simulink model "Lab_2"  (R2017b)
settings: Solver=ode45  StartTime=0.0  StopTime=50  RelTol=1e-10
values from neighbouring files (symbols this model uses):
  I_1 = M/12 * (w^2 + l^2)    (= 0.0153029225)    [main.m]
  I_2 = M/12 * (w^2 + h^2)    (= 0.0314850625)    [main.m]
  I_3 = M/12 * (l^2 + h^2)    (= 0.041787985)    [main.m]
undefined symbols (not defined in the file or in its folder): DCM_0, phi_0, psi_0, theta_0
libraries: sharedutil x1
settings Model: Creator=fcuzzocrea  LastModifiedBy=fcuzzocrea

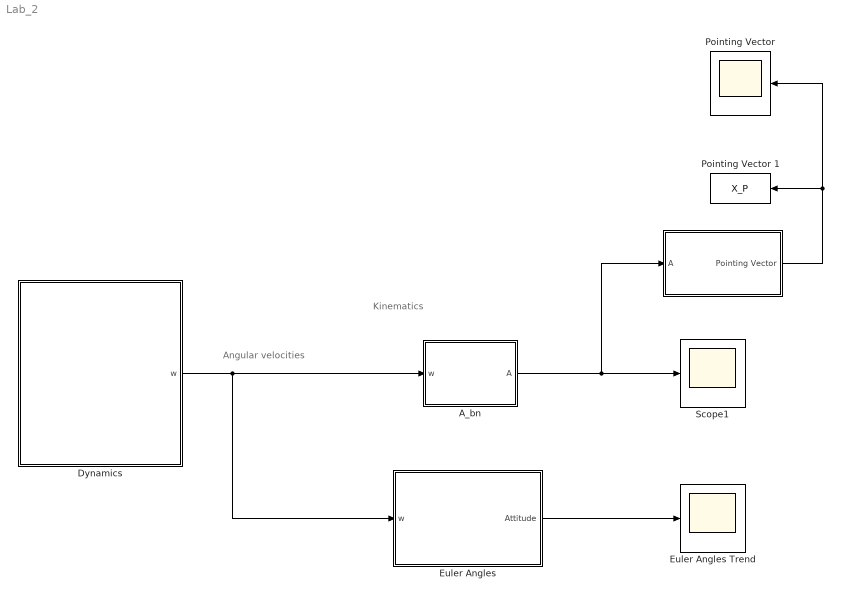
== system Lab_2 ==
  note: Kinematics
  note: Angular velocities
  " " : Subsystem
  A_bn : Subsystem
  "Dynamics " : Subsystem
  "Euler Angles " : Subsystem
  "Euler Angles Trend " : Scope
  Pointing Vector : Scope
  Pointing Vector 1 : ToWorkspace  VariableName=X_P  SampleTime=-1
  Scope1 : Scope
  wires:
  A_bn/1(A) -> " "/1(A), Scope1/1
  "Euler Angles "/1(Attitude) -> "Euler Angles Trend "/1
  "Dynamics "/1(w) -> "Euler Angles "/1(w), A_bn/1(w)
  " "/1("Pointing Vector ") -> Pointing Vector/1, Pointing Vector 1/1

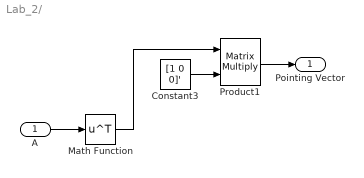
== system Lab_2/  ==
  A : Inport
  Constant3 : Constant  Value=[1 0 0]'  VectorParams1D=off
  Math Function : Math  Operator=transpose  SaturateOnIntegerOverflow=on
  Product1 : Product  Multiplication=Matrix(*)
  "Pointing Vector " : Outport
  wires:
  Constant3/1 -> Product1/2
  Math Function/1 -> Product1/1
  A/1 -> Math Function/1
  Product1/1 -> "Pointing Vector "/1

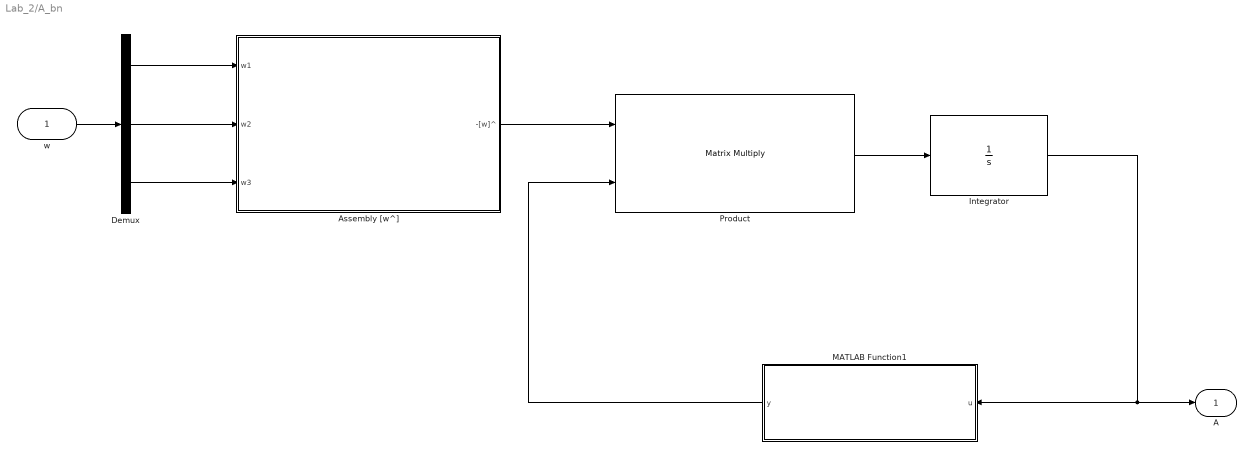
== system Lab_2/A_bn ==
  w : Inport  Unit=rad/s  PortDimensions=3
  "Assembly [w^] " : Subsystem
  Demux : Demux  Outputs=3
  Integrator : Integrator  InitialCondition=DCM_0
  MATLAB Function1 : MATLAB Function  TreatAsAtomicUnit=on
  Product : Product  Multiplication=Matrix(*)
  A : Outport
  wires:
  Product/1 -> Integrator/1
  Integrator/1 -> A/1, MATLAB Function1/1(u)
  w/1 -> Demux/1
  Demux/1 -> "Assembly [w^] "/1(w1)
  Demux/2 -> "Assembly [w^] "/2(w2)
  Demux/3 -> "Assembly [w^] "/3(w3)
  "Assembly [w^] "/1(-[w]^) -> Product/1
  MATLAB Function1/1(y) -> Product/2

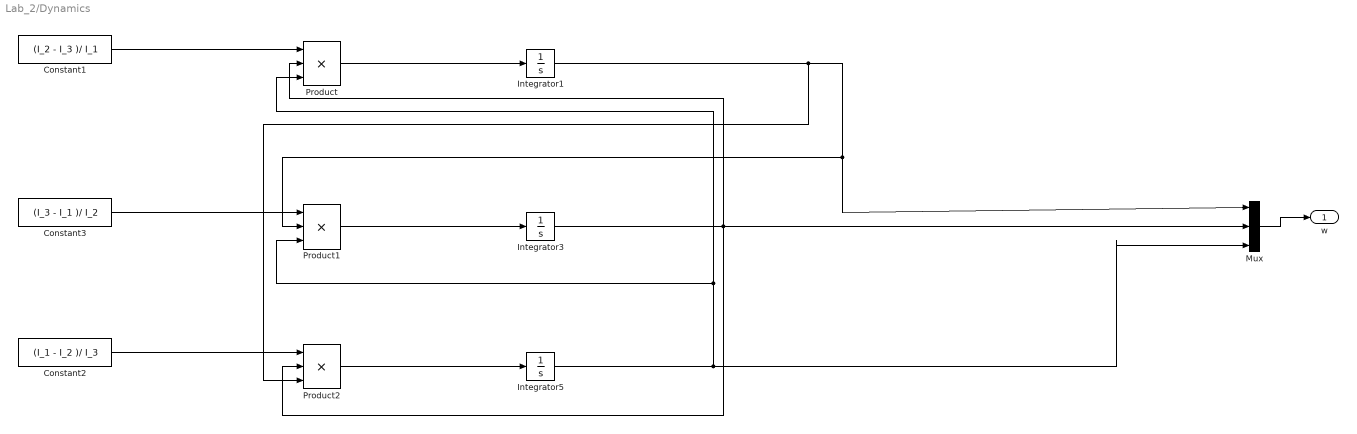
== system Lab_2/Dynamics  ==
  Constant1 : Constant  Value=(I_2 - I_3 )/ I_1
  Constant2 : Constant  Value=(I_1 - I_2 )/ I_3
  Constant3 : Constant  Value=(I_3 - I_1 )/ I_2
  Integrator1 : Integrator
  Integrator3 : Integrator  InitialCondition=0.45
  Integrator5 : Integrator  InitialCondition=0.26
  Mux : Mux  Inputs=3
  Product : Product  Inputs=3
  Product1 : Product  Inputs=3
  Product2 : Product  Inputs=3
  w : Outport
  wires:
  Integrator3/1 -> Mux/2, Product2/2, Product/2
  Integrator5/1 -> Mux/3, Product/3, Product1/3
  Product1/1 -> Integrator3/1
  Product2/1 -> Integrator5/1
  Constant1/1 -> Product/1
  Constant3/1 -> Product1/1
  Constant2/1 -> Product2/1
  Integrator1/1 -> Product2/3, Mux/1, Product1/2
  Product/1 -> Integrator1/1
  Mux/1 -> w/1

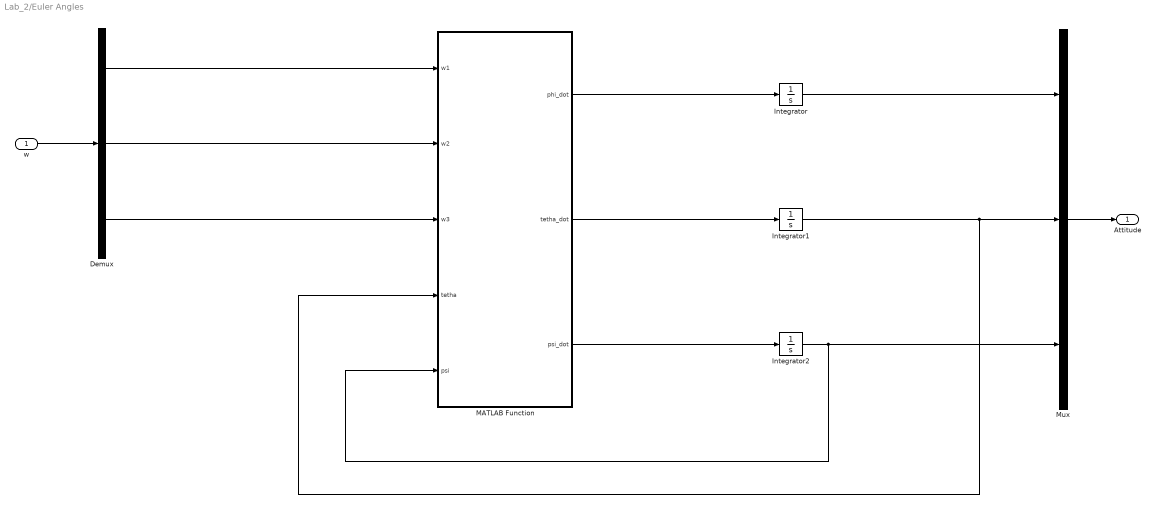
== system Lab_2/Euler Angles  ==
  w : Inport
  Demux : Demux  Outputs=3
  Integrator : Integrator  InitialCondition=phi_0
  Integrator1 : Integrator  InitialCondition=theta_0
  Integrator2 : Integrator  InitialCondition=psi_0
  MATLAB Function : MATLAB Function  TreatAsAtomicUnit=on
  Mux : Mux  Inputs=3
  Attitude : Outport
  wires:
  Demux/1 -> MATLAB Function/1(w1)
  Demux/2 -> MATLAB Function/2(w2)
  Demux/3 -> MATLAB Function/3(w3)
  MATLAB Function/1(phi_dot) -> Integrator/1
  MATLAB Function/2(tetha_dot) -> Integrator1/1
  MATLAB Function/3(psi_dot) -> Integrator2/1
  Integrator/1 -> Mux/1
  Integrator1/1 -> Mux/2, MATLAB Function/4(tetha)
  Mux/1 -> Attitude/1
  Integrator2/1 -> MATLAB Function/5(psi), Mux/3
  w/1 -> Demux/1

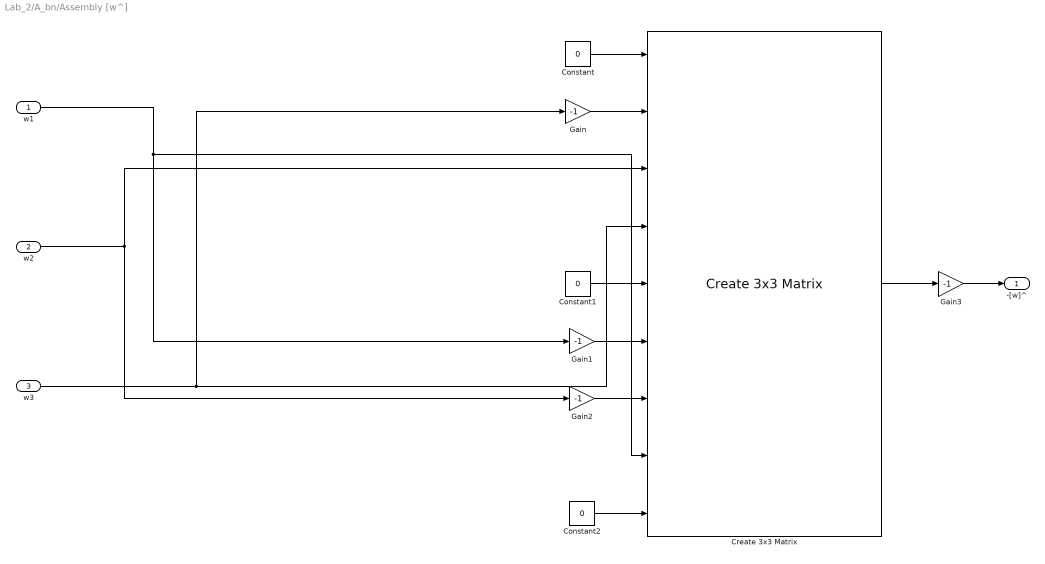
== system Lab_2/A_bn/Assembly [w^]  ==
  w1 : Inport
  w2 : Inport  Port=2
  w3 : Inport  Port=3
  Constant : Constant  Value=0
  Constant1 : Constant  Value=0
  Constant2 : Constant  Value=0
  Create 3x3 Matrix : sharedutil/Create 3x3 Matrix
  Gain{,1..3} (4 alike) : Gain  Gain=-1
  -[w]^ : Outport
  wires:
  Gain2/1 -> Create 3x3 Matrix/7
  Gain1/1 -> Create 3x3 Matrix/6
  w1/1 -> Create 3x3 Matrix/8, Gain1/1
  w3/1 -> Create 3x3 Matrix/4, Gain/1
  Constant1/1 -> Create 3x3 Matrix/5
  Constant2/1 -> Create 3x3 Matrix/9
  Constant/1 -> Create 3x3 Matrix/1
  w2/1 -> Gain2/1, Create 3x3 Matrix/3
  Gain/1 -> Create 3x3 Matrix/2
  Create 3x3 Matrix/1 -> Gain3/1
  Gain3/1 -> -[w]^/1

== matlab function Lab_2/Euler Angles /MATLAB Function ==
  data: phi_dot output; tetha_dot output; psi_dot output; w1 input; w2 input; w3 input; tetha input; psi input
function [phi_dot,tetha_dot, psi_dot] = euler_eqtns(w1,w2,w3, tetha, psi)

% Euler rotations (sequence 123)
phi_dot = 1/cos(tetha)*((w1*cos(psi)-w2*sin(psi)));
tetha_dot = (w2*cos(psi))+(w1*sin(psi));
psi_dot = w3 - ((w1*cos(psi) - w2*sin(psi))*(sin(tetha)/cos(tetha)));

end

== matlab function Lab_2/A_bn/MATLAB Function1 ==
  data: u input; y output
function y = ortonormalize(u)

y = u.*3/2 - u*u'*(u./2);

y = u;

end
